simulink model "RM3_copy2copy"  (R2017b)
settings: Solver=ode4  StartTime=0  StopTime=5000  FixedStep=0.1  MaxStep=0.1  RelTol=1e-3  EnableMultiTasking=on
model workspace (MAT data in the model file):
  p1 = Simulink.Signal
  p1.DataType = 'double'
  p1.Dimensions = -1
  p1.DimensionsMode = 'auto'
  p1.Complexity = 'auto'
  p1.SampleTime = -1
  p1.SamplingMode = 'auto'
values from neighbouring files (symbols this model uses):
  m = min(Out,[],2)    [ContinousControl.m]    (also in RL.m; RealTime_modif22.m)
  N = No*n    (= 60)    [ACTOR_CRITIC & SARSA.m]    (also in TDlearningExampleEforPosting.m)
  num_act = size(action,1)    [CS533DQN_FunctionApproximation.m]    (also in ContinousControl.m; DeepQLearningF.m; HopeGreatRLCode.m; LastFixedEta.m)
  num_state = size(state_spc,1)    [CS533DQN_FunctionApproximation.m]    (also in ContinousControl.m = size(states_space,1); DeepQLearningF.m; HopeGreatRLCode.m; LastFixedEta.m)
  pnum = 1    [ContinousControl.m]    (also in RealTime_modif22.m)
  s = tf('s')    [Fe_extract.m]    (also in InputDataExtraction.m; LetsStartIt.m; SafeLetsStartIt.m; StateExtraction.m)
  states_space = states_spaceP    [ContinousControl.m]    (also in Forward_step.m = states_spaceP([1:9 6*9+1:9*7 15*9+1:9*16 5*9+1:9*6],:); RealTime_modif22.m)
  Ts = states_space( state_idx,2)    [ContinousControl.m]    (also in DeepQLearningF.m = states_space(state_idx,2); EtanStateExtraction.m = TsVec(ts); Forward_step.m = states_space( st_chosen,2); InputDataExtraction.m = TsVec(ts))
  X = YX(:,2:end)    [L2adaptivepredictor.m]
  Y = YX(:,1)    [L2adaptivepredictor.m]
undefined symbols (not defined in the file or in its folder): body, constraint, pto, Z
libraries: nesl_utility x8, sm_lib x5, WECSim_Lib x4, dspstat3 x1, dspindex x1, simulink x1
settings Model: Creator=mlawson  LastModifiedBy=ghleila
settings SolverCC: ZeroCrossControl=DisableAll  AlgebraicLoopSolver=LineSearch  AutoInsertRateTranBlk=on
settings DataIOCC: SaveFormat=Array  SaveOutput=off  SaveTime=off
settings OptimizationCC: LifeSpan=inf  SimCompilerOptimization=on
settings DebuggingCC: UnderspecifiedInitializationDetection=Classic  MergeDetectMultiDrivingBlocksExec=none  SolverPrmCheckMsg=warning  MultiTaskDSMMsg=none  AllowSymbolicDim=off  StateNameClashWarn=warning  SFUnexpectedBacktrackingDiag=warning  SFNoUnconditionalDefaultTransitionDiag=warning  SFExecutionAtInitializationDiag=none
settings HardwareCC: ProdBitPerPointer=32  ProdBitPerSizeT=32  ProdBitPerPtrDiffT=32  ProdLargestAtomicFloat=None  ProdIntDivRoundTo=Undefined  ProdEndianess=Unspecified  ProdWordSize=32  ProdHWDeviceType=32-bit Generic
settings ModelReferenceCC: PropagateSignalLabelsOutOfModel=off
settings CodeAppCC: StateflowObjectComments=on
settings GRTTargetCC: TargetLangStandard=C89/C90 (ANSI)  GeneratePreprocessorConditionals=Disable all
settings ConfigComp: CovMetricSettings=dw  CovHtmlReporting=on  CovSaveCumulativeToWorkspaceVar=on  CovSaveSingleToWorkspaceVar=on  CovExternalEMLEnable=off  CovSFcnEnable=off
settings SimscapeCC: SimscapeNormalizeSystem=off

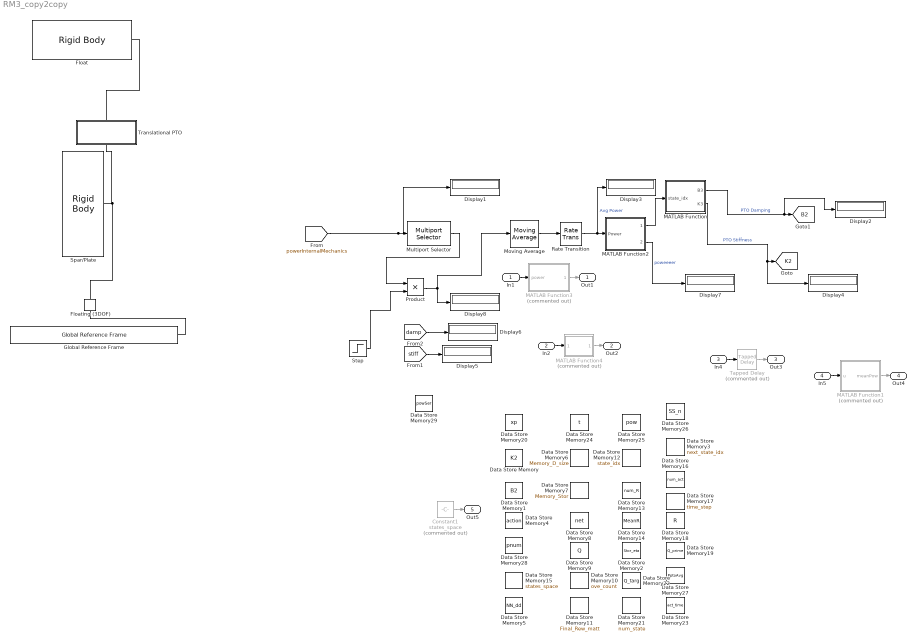
== system RM3_copy2copy ==
  In1 : Inport
  In2 : Inport  Port=2
  In4 : Inport  Port=3
  In5 : Inport  Port=4
  Constant1 : Constant  Commented=on  Value=states_space
  Data Store Memory : DataStoreMemory  DataStoreName=K2  ReadBeforeWriteMsg=warning  WriteAfterWriteMsg=warning  WriteAfterReadMsg=warning  InitialValue=K2  VectorParams1D=off  ShowAdditionalParam=off  OutDataTypeStr=double
  Data Store Memory1 : DataStoreMemory  DataStoreName=B2  ReadBeforeWriteMsg=warning  WriteAfterWriteMsg=warning  WriteAfterReadMsg=warning  InitialValue=B2  VectorParams1D=off  ShowAdditionalParam=off  OutDataTypeStr=double
  Data Store Memory10 : DataStoreMemory  DataStoreName=ove_count  ReadBeforeWriteMsg=warning  WriteAfterWriteMsg=warning  WriteAfterReadMsg=warning  InitialValue=1  VectorParams1D=off  ShowAdditionalParam=off  OutDataTypeStr=double
  Data Store Memory11 : DataStoreMemory  DataStoreName=Final_Rew_matt  ReadBeforeWriteMsg=warning  WriteAfterWriteMsg=warning  WriteAfterReadMsg=warning  InitialValue=zeros(num_state,1)  ShowAdditionalParam=off  OutDataTypeStr=double
  Data Store Memory12 : DataStoreMemory  DataStoreName=state_idx  ReadBeforeWriteMsg=warning  WriteAfterWriteMsg=warning  WriteAfterReadMsg=warning  InitialValue=state_idx  VectorParams1D=off  ShowAdditionalParam=off  OutDataTypeStr=double
  Data Store Memory13 : DataStoreMemory  DataStoreName=num_R  ReadBeforeWriteMsg=warning  WriteAfterWriteMsg=warning  WriteAfterReadMsg=warning  InitialValue=zeros(num_state,1)  VectorParams1D=off  ShowAdditionalParam=off  OutDataTypeStr=double
  Data Store Memory14 : DataStoreMemory  DataStoreName=MeanR  ReadBeforeWriteMsg=warning  WriteAfterWriteMsg=warning  WriteAfterReadMsg=warning  InitialValue=zeros(num_state,1)  VectorParams1D=off  ShowAdditionalParam=off  OutDataTypeStr=double
  Data Store Memory15 : DataStoreMemory  DataStoreName=states_space  ReadBeforeWriteMsg=warning  WriteAfterWriteMsg=warning  WriteAfterReadMsg=warning  InitialValue=states_space  VectorParams1D=off  ShowAdditionalParam=off  OutDataTypeStr=double
  Data Store Memory16 : DataStoreMemory  DataStoreName=num_act  ReadBeforeWriteMsg=warning  WriteAfterWriteMsg=warning  WriteAfterReadMsg=warning  ShowAdditionalParam=off  OutDataTypeStr=double
  Data Store Memory17 : DataStoreMemory  DataStoreName=time_step  ReadBeforeWriteMsg=warning  WriteAfterWriteMsg=warning  WriteAfterReadMsg=warning  ShowAdditionalParam=off  OutDataTypeStr=double
  Data Store Memory18 : DataStoreMemory  DataStoreName=R  ReadBeforeWriteMsg=warning  WriteAfterWriteMsg=warning  WriteAfterReadMsg=warning  InitialValue=zeros(num_state,100)  VectorParams1D=off  ShowAdditionalParam=off  OutDataTypeStr=double
  Data Store Memory19 : DataStoreMemory  DataStoreName=Q_prime  ReadBeforeWriteMsg=warning  WriteAfterWriteMsg=warning  WriteAfterReadMsg=warning  InitialValue=rand(num_state,num_act)  VectorParams1D=off  ShowAdditionalParam=off  OutDataTypeStr=double
  Data Store Memory2 : DataStoreMemory  DataStoreName=Stor_eta  ReadBeforeWriteMsg=warning  WriteAfterWriteMsg=warning  WriteAfterReadMsg=warning  InitialValue=zeros(4000,5)  VectorParams1D=off  ShowAdditionalParam=off  OutDataTypeStr=double
  Data Store Memory20 : DataStoreMemory  DataStoreName=xp  ReadBeforeWriteMsg=warning  WriteAfterWriteMsg=warning  WriteAfterReadMsg=warning  InitialValue=zeros(1,2)  VectorParams1D=off  ShowAdditionalParam=off  OutDataTypeStr=double
  Data Store Memory21 : DataStoreMemory  DataStoreName=num_state  ReadBeforeWriteMsg=warning  WriteAfterWriteMsg=warning  WriteAfterReadMsg=warning  ShowAdditionalParam=off  OutDataTypeStr=double
  Data Store Memory22 : DataStoreMemory  DataStoreName=Q_targ  ReadBeforeWriteMsg=warning  WriteAfterWriteMsg=warning  WriteAfterReadMsg=warning  InitialValue=rand(num_state,num_act)  VectorParams1D=off  ShowAdditionalParam=off  OutDataTypeStr=double
  Data Store Memory23 : DataStoreMemory  DataStoreName=act_time  ReadBeforeWriteMsg=warning  WriteAfterWriteMsg=warning  WriteAfterReadMsg=warning  ShowAdditionalParam=off  OutDataTypeStr=double
  Data Store Memory24 : DataStoreMemory  DataStoreName=t  ReadBeforeWriteMsg=warning  WriteAfterWriteMsg=warning  WriteAfterReadMsg=warning  InitialValue=1  VectorParams1D=off  ShowAdditionalParam=off  OutDataTypeStr=double
  Data Store Memory25 : DataStoreMemory  DataStoreName=pow  ReadBeforeWriteMsg=warning  WriteAfterWriteMsg=warning  WriteAfterReadMsg=warning  InitialValue=zeros(1,5100)  VectorParams1D=off  ShowAdditionalParam=off  OutDataTypeStr=double
  Data Store Memory26 : DataStoreMemory  DataStoreName=SS_n  ReadBeforeWriteMsg=warning  WriteAfterWriteMsg=warning  WriteAfterReadMsg=warning  InitialValue=SS_n  VectorParams1D=off  ShowAdditionalParam=off  OutDataTypeStr=double
  Data Store Memory27 : DataStoreMemory  DataStoreName=PptoAvg  ReadBeforeWriteMsg=warning  WriteAfterWriteMsg=warning  WriteAfterReadMsg=warning  ShowAdditionalParam=off  OutDataTypeStr=double
  Data Store Memory28 : DataStoreMemory  DataStoreName=pnum  ReadBeforeWriteMsg=warning  WriteAfterWriteMsg=warning  WriteAfterReadMsg=warning  ShowAdditionalParam=off  OutDataTypeStr=double
  Data Store Memory29 : DataStoreMemory  DataStoreName=powSer  ReadBeforeWriteMsg=warning  WriteAfterWriteMsg=warning  WriteAfterReadMsg=warning  InitialValue=zeros(1,20*Ts/0.1)  VectorParams1D=off  ShowAdditionalParam=off  OutDataTypeStr=double
  Data Store Memory3 : DataStoreMemory  DataStoreName=next_state_idx  ReadBeforeWriteMsg=warning  WriteAfterWriteMsg=warning  WriteAfterReadMsg=warning  InitialValue=1  ShowAdditionalParam=off  OutDataTypeStr=double
  Data Store Memory4 : DataStoreMemory  DataStoreName=action  ReadBeforeWriteMsg=warning  WriteAfterWriteMsg=warning  WriteAfterReadMsg=warning  InitialValue=action  VectorParams1D=off  ShowAdditionalParam=off  OutDataTypeStr=double
  Data Store Memory5 : DataStoreMemory  DataStoreName=NN_dd  ReadBeforeWriteMsg=warning  WriteAfterWriteMsg=warning  WriteAfterReadMsg=warning  InitialValue=NN_dd  ShowAdditionalParam=off  OutDataTypeStr=double
  Data Store Memory6 : DataStoreMemory  DataStoreName=Memory_D_size  ReadBeforeWriteMsg=warning  WriteAfterWriteMsg=warning  WriteAfterReadMsg=warning  InitialValue=Memory_D_size  VectorParams1D=off  ShowAdditionalParam=off  OutDataTypeStr=double
  Data Store Memory7 : DataStoreMemory  DataStoreName=Memory_Stor  ReadBeforeWriteMsg=warning  WriteAfterWriteMsg=warning  WriteAfterReadMsg=warning  InitialValue=zeros(4000,4+size(states_space,2)+num_act)  ShowAdditionalParam=off  OutDataTypeStr=double
  Data Store Memory8 : DataStoreMemory  DataStoreName=net  ReadBeforeWriteMsg=warning  WriteAfterWriteMsg=warning  WriteAfterReadMsg=warning  VectorParams1D=off  ShowAdditionalParam=off  OutDataTypeStr=double
  Data Store Memory9 : DataStoreMemory  DataStoreName=Q  ReadBeforeWriteMsg=warning  WriteAfterWriteMsg=warning  WriteAfterReadMsg=warning  InitialValue=rand(num_state,num_act)  VectorParams1D=off  ShowAdditionalParam=off  OutDataTypeStr=double
  Display{1..8} (8 alike) : Display
  Float : WECSim_Lib/Body Elements/Rigid Body  body=body(1)
      settings: AttributesFormatString=%<body>
  Floating (3DOF) : WECSim_Lib/Constraints/Floating (3DOF)  constraint=constraint(1)
      settings: AttributesFormatString=%<constraint>
  Global Reference Frame : WECSim_Lib/Frames/Global Reference Frame  waves=waves  simu=simu
  MATLAB Function : MATLAB Function  TreatAsAtomicUnit=on
  MATLAB Function1 : MATLAB Function  Commented=on  TreatAsAtomicUnit=on
  MATLAB Function2 : MATLAB Function  TreatAsAtomicUnit=on
  MATLAB Function3 : MATLAB Function  Commented=on  TreatAsAtomicUnit=on
  MATLAB Function4 : MATLAB Function  Commented=on  TreatAsAtomicUnit=on
  Moving Average : dspstat3/Moving Average  Method=Sliding window  SpecifyWindowLength=on  WindowLength=20*Ts/0.1  ForgettingFactor=0.9  SimulateUsing=Code generation
  Multiport Selector : dspindex/Multiport Selector  rowsOrCols=Rows  idxCellArray={ 3}  idxErrMode=Clip Index
  Product : Product
  Rate Transition : RateTransition  OutPortSampleTime=20*Ts
  Spar/Plate : WECSim_Lib/Body Elements/Rigid Body  body=body(2)
      settings: AttributesFormatString=%<body>
  Step : Step  SampleTime=20*pnum*10
  Tapped Delay : simulink/Discrete/Tapped Delay  Commented=on  vinit=0.0  samptime=-1  NumDelays=4  DelayOrder=Oldest  includeCurrent=off
  Translational PTO : Subsystem  AncestorBlock=WECSim_Lib/PTOs/Translational PTO  mask(PTO){pto=pto(1)}
      mask prompts: pto "PTO Name:"
      mask help:
      | Constraints the follower to translational motion relative to the base, in
      | the PTO's Z-direction and adds PTO stiffness and damping.
      |
      |
      | The variable name input below must be 'pto(i)' where i=1,2,...
      | pto(i) must be defined in the input file with the following fields:
      |
      |     .name (required)
      |             String.
      |             PTO name. Must comply with Matlab's variable naming rules.
      |     .loc (optional)
      |             3x1 vector [x y z] in meters.
      |             PTO location. Default = [0 0 0]
      |     .k (optional)
      |             Float.
      |             PTO linear spring stiffness. Default = 0
      |     .c (optional)
      |             Float.
      |             PTO linear damping coefficient. Default = 0
      |     .orientation.z (optional)
      |             3x1 vector [x y z].
      |             Direction of the PTO's Z-coordinate. Default = [0 0 1]
      |     .orientation.y (optional)
      |             3x1 vector [x y z].
      |             Direction of the PTO's Y-coordinate. Default = [0 1 0]
      mask init:
      | if exist('pto','var')
      |     h=[gcb '/output'];
      |     responseName=['pto' num2str(pto.ptoNum) '_out'];
      |     set_param(h,'VariableName',responseName);
      | end
      | 
      | pto.checkLoc('W');
      settings: AttributesFormatString=%<pto>
      mask Help:
      | Constraints the follower to translational motion relative to the base, in
      | the PTO's Z-direction and adds PTO stiffness and damping.
      | 
      | 
      | The variable name input below must be 'pto(i)' where i=1,2,...
      | pto(i) must be defined in the input file with the following fields:
      | 
      |     .name (required)
      |             String.
      |             PTO name. Must comply with Matlab's variable naming rules.
      |     .loc (optional)
      |             3x1 vector [x y z] in meters.
      |             PTO location. Default = [0 0 0]
      |     .k (optional)
      |             Float.
      |             PTO linear spring stiffness. Default = 0
      |     .c (optional)
      |             Float.
      |             PTO linear damping coefficient. Default = 0
      |     .orientation.z (optional)
      |             3x1 vector [x y z].
      |             Direction of the PTO's Z-coordinate. Default = [0 0 1]
      |     .orientation.y (optional)
      |             3x1 vector [x y z].
      |             Direction of the PTO's Y-coordinate. Default = [0 1 0]
  Out1 : Outport
  Out2 : Outport  Port=2
  Out3 : Outport  Port=3
  Out4 : Outport  Port=4
  Out5 : Outport  Port=5
  tag scope: B2=global, K2=global
  wires:
  In4/1 -> Tapped Delay/1
  MATLAB Function4/1(powSer1) -> Out2/1
  In2/1 -> MATLAB Function4/1(WholepowSer)
  MATLAB Function/1(B3) -> Display2/1, [B2]  "PTO Damping"
  [damp] -> Display6/1
  In5/1 -> MATLAB Function1/1(u)
  Tapped Delay/1 -> Out3/1
  Multiport Selector/1 -> Product/1
  MATLAB Function2/1(state_idx1) -> MATLAB Function/1(state_idx)
  Step/1 -> Product/2
  [stiff] -> Display5/1
  Moving Average/1 -> Rate Transition/1
  Constant1/1 -> Out5/1
  MATLAB Function3/1(PowSum) -> Out1/1
  MATLAB Function1/1(meanPow) -> Out4/1
  In1/1 -> MATLAB Function3/1(power)
  [powerInternalMechanics] -> Display1/1, Multiport Selector/1
  MATLAB Function/2(K3) -> Display4/1, [K2]  "PTO Stiffness"
  Rate Transition/1 -> Display3/1, MATLAB Function2/1(Power)  "Avg Power"
  Product/1 -> Display8/1, Moving Average/1
  MATLAB Function2/2(PptoAvg1) -> Display7/1  "poweeeer"
  connections:
  Translational PTO/RConn1 -- Floating (3DOF)/RConn1 -- Spar/Plate/RConn1
  Floating (3DOF)/LConn1 -- Global Reference Frame/RConn1
  Translational PTO/LConn1 -- Float/RConn1

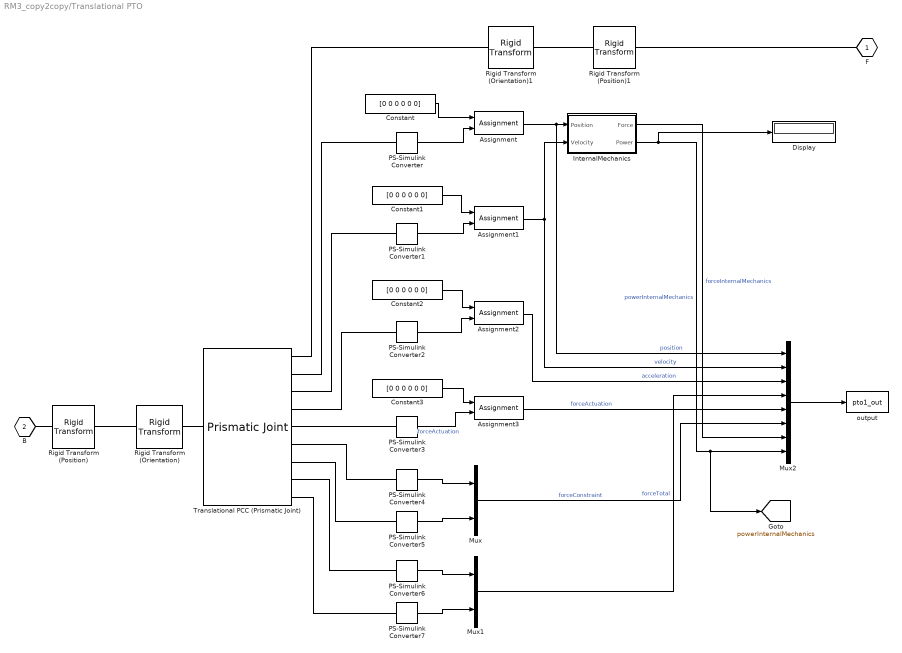
== system RM3_copy2copy/Translational PTO ==
  Assignment{,1..3} (4 alike) : Assignment  IndexOptions=Index vector (dialog)  Indices=3  OutputSizes=1
  Constant{,1..3} (4 alike) : Constant  Value=[0 0 0 0 0 0]
  Display : Display
  InternalMechanics : Subsystem
  Mux : Mux  Inputs=2
  Mux1 : Mux  Inputs=2
  Mux2 : Mux  Inputs=8
  PS-Simulink Converter{,1..7} (8 alike) : nesl_utility/PS-Simulink Converter  PhysicalDomain=network_engine_domain  SubClassName=ps_output  LeftPortType=input  RightPortType=output  PseudoPeriodic=off  Frequencies=[]  Unit=1  AffineConversion=off
  Rigid Transform (Position) : sm_lib/Frames and Transforms/Rigid Transform  TranslationMethod=Cartesian  TranslationStandardOffset=0  TranslationLengthUnit=m  TranslationStandardAxis=+Z  TranslationCartesianOffset=pto.initDisp.initLinDisp + pto.loc  TranslationROffset=0  TranslationROffsetUnits=m  TranslationZOffset=0  TranslationZOffsetUnits=m  TranslationThetaOffset=0  TranslationThetaOffsetUnits=deg  RotationMethod=None  RotationAngleUnits=rad  RotationStandardAxis=+Y  RotationAngle=0  RotationArbitraryAxis=[0 1 0]  FollAlignAxisA=+X  BaseAlignAxisA=+Y  FollAlignAxisB=+Y  BaseAlignAxisB=+Z  RotationSequenceAxes=FollowerAxes  RotationSequence=XYX  RotationSequenceAngles=[0 0 0]  RotationSequenceAnglesUnits=deg  RotationMatrix=[1 0 0; 0 1 0; 0 0 1]
  Rigid Transform (Position)1 : sm_lib/Frames and Transforms/Rigid Transform  TranslationMethod=Cartesian  TranslationStandardOffset=0  TranslationLengthUnit=m  TranslationStandardAxis=+Z  TranslationCartesianOffset=pto.initDisp.initLinDisp + pto.loc  TranslationROffset=0  TranslationROffsetUnits=m  TranslationZOffset=0  TranslationZOffsetUnits=m  TranslationThetaOffset=0  TranslationThetaOffsetUnits=deg  RotationMethod=None  RotationAngleUnits=rad  RotationStandardAxis=+Y  RotationAngle=0  RotationArbitraryAxis=[0 1 0]  FollAlignAxisA=+X  BaseAlignAxisA=+Y  FollAlignAxisB=+Y  BaseAlignAxisB=+Z  RotationSequenceAxes=FollowerAxes  RotationSequence=XYX  RotationSequenceAngles=[0 0 0]  RotationSequenceAnglesUnits=deg  RotationMatrix=[1 0 0; 0 1 0; 0 0 1]
  Rigid Transform (Orientation) : sm_lib/Frames and Transforms/Rigid Transform  TranslationMethod=None  TranslationStandardOffset=0  TranslationLengthUnit=m  TranslationStandardAxis=+Z  TranslationCartesianOffset=0  TranslationROffset=0  TranslationROffsetUnits=m  TranslationZOffset=0  TranslationZOffsetUnits=m  TranslationThetaOffset=0  TranslationThetaOffsetUnits=deg  RotationMethod=RotationMatrix  RotationAngleUnits=rad  RotationStandardAxis=+Y  RotationAngle=0  RotationArbitraryAxis=[0 1 0]  FollAlignAxisA=+X  BaseAlignAxisA=+Y  FollAlignAxisB=+Y  BaseAlignAxisB=+Z  RotationSequenceAxes=FollowerAxes  RotationSequence=XYX  RotationSequenceAngles=[0 0 0]  RotationSequenceAnglesUnits=deg  RotationMatrix=pto.orientation.rotationMatrix
  Rigid Transform (Orientation)1 : sm_lib/Frames and Transforms/Rigid Transform  TranslationMethod=None  TranslationStandardOffset=0  TranslationLengthUnit=m  TranslationStandardAxis=+Z  TranslationCartesianOffset=0  TranslationROffset=0  TranslationROffsetUnits=m  TranslationZOffset=0  TranslationZOffsetUnits=m  TranslationThetaOffset=0  TranslationThetaOffsetUnits=deg  RotationMethod=RotationMatrix  RotationAngleUnits=rad  RotationStandardAxis=+Y  RotationAngle=0  RotationArbitraryAxis=[0 1 0]  FollAlignAxisA=+X  BaseAlignAxisA=+Y  FollAlignAxisB=+Y  BaseAlignAxisB=+Z  RotationSequenceAxes=FollowerAxes  RotationSequence=XYX  RotationSequenceAngles=[0 0 0]  RotationSequenceAnglesUnits=deg  RotationMatrix=pto.orientation.rotationMatrix
  Translational PCC (Prismatic Joint) : sm_lib/Joints/Prismatic Joint  SenseConstraintForce=on  SenseConstraintForceX=off  SenseConstraintForceY=off  SenseConstraintForceZ=off  SenseConstraintTorque=on  SenseConstraintTorqueX=off  SenseConstraintTorqueY=off  SenseConstraintTorqueZ=off  SenseTotalForce=on  SenseTotalForceX=off  SenseTotalForceY=off  SenseTotalForceZ=off  SenseTotalTorque=on  SenseTotalTorqueX=off  SenseTotalTorqueY=off  SenseTotalTorqueZ=off  CompositeWrenchDir=BaseOnFollower  CompositeWrenchFrame=BaseFrame  EquilibriumPosition=0  EquilibriumPositionUnits=m  SpringStiffness=pto.k  SpringStiffnessUnits=N/m  DampingCoefficient=pto.c  DampingCoefficientUnits=N/(m/s)  TorqueActuationMode=NoTorque  MotionActuationMode=ComputedMotion  SensePosition=on  SenseVelocity=on  SenseAcceleration=on  SenseTorqueForce=on  PositionTargetSpecify=off  PositionTargetPriority=High  PositionTargetValue=0  PositionTargetValueUnits=m  VelocityTargetSpecify=off  VelocityTargetPriority=High  VelocityTargetValue=0  VelocityTargetValueUnits=m/s
  output : ToWorkspace  VariableName=pto1_out  SaveFormat=Structure With Time  SampleTime=-1
      settings: Decimation=round(simu.dtOut/simu.dt,0)
  F : PMIOPort  Port=1  Side=Left
  B : PMIOPort  Port=2  Side=Right
  tag scope: powerInternalMechanics=global
  wires:
  PS-Simulink Converter3/1 -> Assignment3/2  "forceActuation"
  Constant3/1 -> Assignment3/1
  InternalMechanics/2(Power) -> Display/1, [powerInternalMechanics], Mux2/8  "powerInternalMechanics"
  InternalMechanics/1(Force) -> Mux2/7  "forceInternalMechanics"
  PS-Simulink Converter2/1 -> Assignment2/2
  Constant2/1 -> Assignment2/1
  PS-Simulink Converter1/1 -> Assignment1/2
  Constant1/1 -> Assignment1/1
  PS-Simulink Converter/1 -> Assignment/2
  Constant/1 -> Assignment/1
  Assignment2/1 -> Mux2/3  "acceleration"
  Assignment1/1 -> InternalMechanics/2(Velocity), Mux2/2  "velocity"
  Assignment/1 -> InternalMechanics/1(Position), Mux2/1  "position"
  Assignment3/1 -> Mux2/5  "forceActuation"
  PS-Simulink Converter7/1 -> Mux1/2
  PS-Simulink Converter6/1 -> Mux1/1
  PS-Simulink Converter5/1 -> Mux/2
  PS-Simulink Converter4/1 -> Mux/1
  Mux1/1 -> Mux2/4  "forceTotal"
  Mux/1 -> Mux2/6  "forceConstraint"
  Mux2/1 -> output/1
  connections:
  Rigid Transform (Position)/RConn1 -- Rigid Transform (Orientation)/LConn1
  Rigid Transform (Position)1/RConn1 -- Rigid Transform (Orientation)1/LConn1
  Rigid Transform (Orientation)/RConn1 -- Translational PCC (Prismatic Joint)/LConn1
  Translational PCC (Prismatic Joint)/RConn6 -- PS-Simulink Converter4/LConn1
  Translational PCC (Prismatic Joint)/RConn2 -- PS-Simulink Converter/LConn1
  Translational PCC (Prismatic Joint)/RConn8 -- PS-Simulink Converter6/LConn1
  Rigid Transform (Position)1/LConn1 -- F/RConn1
  Translational PCC (Prismatic Joint)/RConn3 -- PS-Simulink Converter1/LConn1
  Translational PCC (Prismatic Joint)/RConn7 -- PS-Simulink Converter5/LConn1
  Translational PCC (Prismatic Joint)/RConn4 -- PS-Simulink Converter2/LConn1
  Rigid Transform (Orientation)1/RConn1 -- Translational PCC (Prismatic Joint)/RConn1
  Translational PCC (Prismatic Joint)/RConn9 -- PS-Simulink Converter7/LConn1
  Translational PCC (Prismatic Joint)/RConn5 -- PS-Simulink Converter3/LConn1
  Rigid Transform (Position)/LConn1 -- B/RConn1

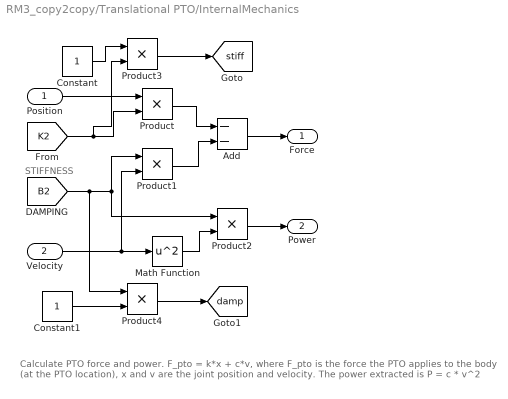
== system RM3_copy2copy/Translational PTO/InternalMechanics ==
  note: STIFFNESS
  note: Calculate PTO force and power.
      |
      | F_pto  = k*x + c*v,
      | where F_pto is the force the PTO applies to the body (at the PTO location), x and v are the joint position and velocity.
      |
      | The power extracted is
      | P = c * v^2
  Position : Inport
  Velocity : Inport  Port=2
  Add : Sum  Inputs=--
  Constant : Constant
  Constant1 : Constant
  Math Function : Math  Operator=square  SaturateOnIntegerOverflow=on
  Product{,1..4} (5 alike) : Product  Inputs=**
  Force : Outport
  Power : Outport  Port=2
  tag scope: damp=global, stiff=global
  wires:
  Product1/1 -> Add/2
  Product/1 -> Add/1
  Math Function/1 -> Product2/2
  Add/1 -> Force/1
  Position/1 -> Product/1
  [K2] -> Product3/2, Product/2
  Velocity/1 -> Product1/2, Math Function/1
  Product2/1 -> Power/1
  [B2] -> Product4/1, Product1/1, Product2/1
  Constant/1 -> Product3/1
  Product3/1 -> [stiff]
  Constant1/1 -> Product4/2
  Product4/1 -> [damp]

== matlab function RM3_copy2copy/MATLAB Function ==
  data: ove_count data_store_memory; action data_store_memory; xp data_store_memory; B2 data_store_memory; K2 data_store_memory; Stor_eta data_store_memory; states_space data_store_memory; num_R data_store_memory; MeanR data_store_memory; R data_store_memory; Final_Rew_matt data_store_memory; NN_dd data_store_memory; Memory_D_size data_store_memory; Memory_Stor data_store_memory; Q_prime data_store_memory; Q_targ data_store_memory; Q data_store_memory; B3 output; K3 output; SS_n data_store_memory; state_idx input; next_state_idx data_store_memory
function [B3,K3]=fcn1(state_idx)

global ove_count action B2 K2 Stor_eta Q states_space next_state_idx 
%B2 K2 act_time  SS_n  NN_dd Memory_D_size Memory_Stor  Q ove_count...
 %     state_idx  states_space action Stor_eta num_R MeanR  Q_targ num_state num_act time_step Q_prime  R Final_Rew_matt;


%  pow=power(end-act_time/time_step:end);
% 
% mean_six_pow=mean(pow);
%PptoAvg=mean_six_pow;





%% initial state
    
   % for ove_count1=1:1500
  
        coder.extrinsic('num2str','datasample','get_param','feedforwardnet','train'); 
        
      
   
        disp(['iteration: ' num2str(ove_count)]);
        
        %     if ove_count>=500
        %
        %          gamma=gamma_int/((ove_count)^-0.06);
        %     else
        %
        %         gamma=gamma_int;
        %
        %     end
         
          if ove_count>=150
            
            epsilon=0;
           % opts.StepRatio = 0.01;
               
                else  
            
            epsilon=1;
           % opts.StepRatio = 0.1;
            
        end
        
        %% taking an action
        
            r=rand; % get 1 uniform random number
        
            x=sum(r>=cumsum([0, 1-epsilon, epsilon])); % check it to be in which probability area
            % choose either explore or exploit
        
            if x == 1   % exploit
        
                [~,umax]=max(Q(state_idx,:));
        
                % [~,umax]=max(V(state_idx,1));
        
                current_action = action(umax,:);
        
            else        % explore
        

      % action_idx=zeros(1,1); 
        
        current_action=datasample(action,1); % choose 1 action randomly (uniform random distribution)
            end

       B2=current_action(1,1);
%        
         K2=current_action(1,2);
         
         action_idx = find(action(:,1)==B2 & action(:,2)==K2); % id of the chosen action
%         
       %         %% storing eta for reconstruction 
%         
       
Stor_eta(ove_count,1)=state_idx;
%         %Stor_eta(ove_count,2)=irreg_eta_idx

%[d f]=size(int(action_idx))
action_idx=action_idx(1,1);
        
      Stor_eta(ove_count,2)=action_idx;
      
      %% next state
        st_chosen=double(0); 
        st_chosen=datasample(1:size(states_space,1),1); % choose 1 action randomly (uniform random distribution)

        Height =states_space( st_chosen,1);           %m         %Amplitude of the waves
       
        Ts =states_space( st_chosen,2);             %s         %Significant period of the Wave

        next_state_idx1=0;
      next_state_idx1=find(states_space(:,1)==Height & states_space(:,2)==Ts & states_space(:,3)==B2 & states_space(:,4)==K2);
       next_state_idx=next_state_idx1(1,1);

gh=next_state_idx
        
        %% produce eta for the current state
        
% %         tsim_ove=60*Ts;  %%
% %         delta_t=0.01;
% %         StepT_SIM=0.01;

        %% next_state
%         
%         Height =states_space( state_idx,1);           %m         %Amplitude of the waves
%         
%         Ts =states_space( state_idx,2);
%         
%         next_stPrimee_idx=find(states_space(:,1)==Height & states_space(:,2)==Ts & states_space(:,3)==B2 & states_space(:,4)==K2);
% 
% 
%         
% % %         FeWithTime=[];
% % %         
% % %         FeWithTime=makeEtaFe(Height,Ts,tsim_ove,delta_t,A1,B1,K1);
% % %         
% % %         [PptoAvg]=TstSimulatorF(FeWithTime,A1,B1,K1,B2,K2,tsim_ove,StepT_SIM,state_idx);   % initiaL STATE
% % %       
% % %         wecSimInputFile;
% % %         wecSim;
% % %        %%% userDefinedFunctions
% % %         PP=output.ptos.powerInternalMechanics;
% % %         
% % %         mean_six_pow=mean(PP);
% % %         PptoAvg=mean_six_pow(1,3)
% % %         
% % %         hg(ove_count1)=PptoAvg;
% 
%         %% next state
%         st_chosen=double(0); 
%         st_chosen=datasample(1:size(states_space,1),1); % choose 1 action randomly (uniform random distribution)
%         
%         
%         Height_prime =states_space( st_chosen,1);           %m         %Amplitude of the waves
%         Ts_prime =states_space( st_chosen,2);             %s         %Significant period of the Wave
%         
%         next_state_idx=find(states_space(:,1)==Height_prime & states_space(:,2)==Ts_prime & states_space(:,3)==B2 & states_space(:,4)==K2);
%         
%         
%         %% allocating power
%         num_R(next_stPrimee_idx)=num_R(next_stPrimee_idx)+1;
%         next_reward=(PptoAvg/(Height^2)); %% normalized reward
%         %num_R(state_idx)=2;
%         R(next_stPrimee_idx,num_R(next_stPrimee_idx))=next_reward
%         Height=states_space(next_stPrimee_idx,1);
%         Height=Height(1,1);
%         next_state_idx;
%         
%         Period=states_space(next_stPrimee_idx,2);
%         Period=Period(1,1);
%         
%        
%         R_idx=find(states_space(:,1)==Height& states_space(:,2)==Period);
%         
%         MeanR(R_idx,1)=sum(R(R_idx,:),2)./num_R(R_idx) % mean
%         
%         % MaxR=max(max(R(R_idx)));
%         
%         MaxR=max(MeanR(R_idx));
%         
%                
%         Final_Rew_matt(R_idx)=MeanR(R_idx,1)/MaxR;
%         
%         Final_Rew=Final_Rew_matt(next_stPrimee_idx);
%         
%         Final_Rew=(Final_Rew)^5;
%         
% % %         if (PptoAvg/1e06)<=0.1
% % %             Final_Rew=-1;
% % %         end
%         
%         %     if ove_count>150
%         %
%         %         if Final_Rew==1
%         %         Final_Rew=10;
%         %         end
%         %     end
%         
%        % Stor_eta(ove_count,3)=(All_params3(1,1)); Stor_eta(ove_count,4)=(All_params3(1,2)); 
%        %%% so what
%         Stor_eta(ove_count,3)=B2;
%         Stor_eta(ove_count,4)=K2;  Stor_eta(ove_count,5)=PptoAvg;
% %         
%         
%    
%         %% storing features
%         
%        % All_features(ove_count,:)=All_params3;  %%% to get an idea about the max of each parameter
%         
%         disp(['current state : ' num2str(state_idx) ' next state : ' num2str(next_state_idx) ' taken action : ' num2str(action(action_idx,:))]);
%         
%         disp([' next reward : ' num2str(Final_Rew)]);
%         
%         %% neural network part
%         
%         
%         if ove_count> 10  %% start traing network
%             
%                         %% droping off very old data
%             
%             if ove_count>Memory_D_size %% dropoff
%                 
%                 In=Memory_Stor(ove_count-Memory_D_size:ove_count-1,5:8);
%                 
%                 Output=Memory_Stor(ove_count-Memory_D_size:ove_count-1,9:end);
%                 
%                 nodes = [size(In,2) size(action,1)];
%                 
%             else
%                 
%                 In=Memory_Stor(1:ove_count-1,5:8);
%                 
%                 Output=Memory_Stor(1:ove_count-1,9:end);
%                 
%                 nodes = [size(In,2) size(action,1)];
%                 
%             end
%             
%            % % % % %             
% % % % %             In=Memory_Stor(:,5:8);
% % % % %             
% % % % %             Output=Memory_Stor(:,9:end);
% % % % %             
%             
%                 Out=[];
%                 Out=Output;
%                 m = min(Out,[],2);  
%                 range = max(Out,[],2) - m;      
%                Out1=bsxfun(@minus,Out,m);
%                Out=bsxfun(@rdivide,Out1,range) ;
%             
%                 Input=[];
%                 Input=In;
%                 m11 = min(Input);
%                range1 = max(Input) - m11;
%                Input=bsxfun(@minus,Input,m11);
%                Input=bsxfun(@rdivide,Input,range1) ;
%                
%            
%                %% correction for one sea state
%                 Input(:,1:2) =ones(size(Input,1),2);
%             
%             net = feedforwardnet([5]);
%             [net,tr] = train(net,Input',Out');
% %             
% %             
%             y_prime= net(SS_n(next_state_idx,:)');
%             Q_prime(next_state_idx,:) =y_prime';
%             
%             
%         
%             
%             
% %             % % % %
% % % dnn=[];
% % %                 [dnn,out_est,rmse]=DNNf(Input,Output,nodes,opts);
% % %             Input;
% % %                 g=v2h(dnn, SS_n(next_state_idx,:));
% % %             
% % %                Q_prime(next_state_idx,:) = v2h(dnn, SS_n(next_state_idx,:));
% 
% %ghk=Final_Rew+gamma*max(Q_prime(next_state_idx,:)); % update q values
%            
%             sec_part=Q_prime(next_state_idx,:);
%             sec_part=sec_part(1,:);
%             ghk=Final_Rew+gamma*max(sec_part);
%             ghk=ghk(1,1);
%            Q_targ(state_idx,action_idx)=ghk; % update q values
%             
%             target=Q;
%             Q_prev=Q;
%             
%             target(state_idx,action_idx)=Q_targ(state_idx,action_idx); %%% update target
%             Memory_Stor(ove_count,:)=[state_idx,action_idx,Final_Rew,next_state_idx,states_space(state_idx,:),target(state_idx,:)];
% result=[state_idx,action_idx,Final_Rew]
%             %% training NN with recent data
%             %        [dnn,out_est,rmse]=DNNf(Input,Output,nodes,opts);
%             
%           else
%             % Q_prev=Q;
%             
%            % Q(state_idx,action_idx)=Q(state_idx,action_idx)+alpha*(Final_Rew+gamma*max(Q(next_state_idx,:))-Q(state_idx,action_idx));
%            gh=Q(next_state_idx,:);
%            MaxQ=max(gh(1,:));
%             QQ=Q(state_idx,action_idx);
%             Q3=gamma*MaxQ-Q(state_idx,action_idx);
%             Q_final=Q(state_idx,action_idx)+alpha*(Final_Rew+Q3);
%             Q(state_idx,action_idx)=Q_final(1,1);
%           %  Q(state_idx,action_idx)=Q(state_idx,action_idx)+alpha*(Final_Rew+gamma*max(Q(next_state_idx,:))-Q(state_idx,action_idx));
%             target=Q;
%             
%             Memory_Stor(ove_count,:)=[state_idx,action_idx,Final_Rew,next_state_idx,states_space(state_idx,:),target(state_idx,:)];
%         end
%         
%         %% checking the convergence of  Q function
%         
%         Q=target;
%         
%         % dif(ove_count)=norm(target(:,:)-Q_prev(:,:),Inf);
%         
%         ove_count=ove_count+1;
%         next_state_idx=next_state_idx(1,1);
%         
%         state_idx=next_state_idx;
%         
%    % end
        

B3=B2
K3=K2
        h=1;
        
        
       % d=xp(1,2)

== matlab function RM3_copy2copy/MATLAB Function1 ==
  settings: updateMethod=DISCRETE
  data: u input; t data_store_memory; pow data_store_memory; meanPow output
function meanPow=fcn(u)

%codegen

global t pow
%coder.varsize('k',[1 5000]);

 coder.extrinsic('average')
 k=zeros(1,t);
          pow(1,t)=u(3,:);
          k=pow(1,1:t);
          meanPow=0;
          meanPow=mean(k(1,:));
  
          t=t+1;
%         PptoAvg=mean_six_pow(1,3);

== matlab function RM3_copy2copy/MATLAB Function2 ==
  data: ove_count data_store_memory; action data_store_memory; xp data_store_memory; B2 data_store_memory; K2 data_store_memory; Stor_eta data_store_memory; state_idx data_store_memory; states_space data_store_memory; num_R data_store_memory; MeanR data_store_memory; R data_store_memory; Final_Rew_matt data_store_memory; NN_dd data_store_memory; Memory_D_size data_store_memory; Memory_Stor data_store_memory; Q_prime data_store_memory; Q_targ data_store_memory; Q data_store_memory; Power input; state_idx1 output; SS_n data_store_memory; next_state_idx data_store_memory; PptoAvg data_store_memory; PptoAvg1 output; pnum data_store_memory
function [state_idx1,PptoAvg1] =fcn1(Power)

global ove_count action B2 K2 Stor_eta states_space num_R MeanR state_idx R Final_Rew_matt...
    NN_dd Memory_D_size Memory_Stor Q_prime Q_targ Q SS_n next_state_idx PptoAvg pnum
%B2 K2 act_time  SS_n  NN_dd Memory_D_size Memory_Stor  Q ove_count...
%     state_idx  states_space action Stor_eta num_R MeanR  Q_targ num_state num_act time_step Q_prime  R Final_Rew_matt;


pnum=pnum+1; %set the p1 to zero for next iters

Ts=10; %%% should be global
num=20*Ts/0.1;  %% should be global
%Power=Power/num;

%PptoAvg=Power-PptoAvg;
PptoAvg=Power;

PptoAvg1=PptoAvg;

%  pow=power(end-act_time/time_step:end);
%
% mean_six_pow=mean(pow);
%PptoAvg=mean_six_pow;
%% initial state

% for ove_count1=1:1500

coder.extrinsic('num2str','datasample','get_param','feedforwardnet','train');


if ove_count>=150
    
    gamma=0.9;
    % opts.StepRatio = 0.01;
else
    
    gamma=0.6;
    % opts.StepRatio = 0.1;
    
end


if ove_count>=150
    
    alpha=0.6;
    
else
    
    alpha=0.4;
    
end




%         %% taking an action
%
%             r=rand; % get 1 uniform random number
%
%             x=sum(r>=cumsum([0, 1-epsilon, epsilon])); % check it to be in which probability area
%             % choose either explore or exploit
%
%             if x == 1   % exploit
%
%                 [~,umax]=max(Q(state_idx,:));
%
%                 % [~,umax]=max(V(state_idx,1));
%
%                 current_action = action(umax,:);
%
%             else        % explore
%
%
%       % action_idx=zeros(1,1);
%
%         current_action=datasample(action,1); % choose 1 action randomly (uniform random distribution)
%             end
%
%        B2=current_action(1,1);
% %
%          K2=current_action(1,2);
%
%          action_idx = find(action(:,1)==B2 & action(:,2)==K2); % id of the chosen action
% %
%        %         %% storing eta for reconstruction
% %
%
% Stor_eta(ove_count,1)=state_idx;
% %         %Stor_eta(ove_count,2)=irreg_eta_idx
%
% %[d f]=size(int(action_idx))
% action_idx=action_idx(1,1);
%
%       Stor_eta(ove_count,2)=action_idx;
%
%% produce eta for the current state

% %         tsim_ove=60*Ts;  %%
% %         delta_t=0.01;
% %         StepT_SIM=0.01;

%% next_state



action_idx = find(action(:,1)==B2 & action(:,2)==K2);

Height =states_space( next_state_idx,1);           %m         %Amplitude of the waves

Ts =states_space( next_state_idx,2);

% next_stPrimee_idx=find(states_space(:,1)==Height & states_space(:,2)==Ts & states_space(:,3)==B2 & states_space(:,4)==K2);



% %         FeWithTime=[];
% %
% %         FeWithTime=makeEtaFe(Height,Ts,tsim_ove,delta_t,A1,B1,K1);
% %
% %         [PptoAvg]=TstSimulatorF(FeWithTime,A1,B1,K1,B2,K2,tsim_ove,StepT_SIM,state_idx);   % initiaL STATE
% %
% %         wecSimInputFile;
% %         wecSim;
% %        %%% userDefinedFunctions
% %         PP=output.ptos.powerInternalMechanics;
% %
% %         mean_six_pow=mean(PP);
% %         PptoAvg=mean_six_pow(1,3)
% %
% %         hg(ove_count1)=PptoAvg;

%% next state
%         st_chosen=double(0);
%         st_chosen=datasample(1:size(states_space,1),1); % choose 1 action randomly (uniform random distribution)
%
%
%         Height_prime =states_space( st_chosen,1);           %m         %Amplitude of the waves
%         Ts_prime =states_space( st_chosen,2);             %s         %Significant period of the Wave
%
%         next_state_idx=find(states_space(:,1)==Height_prime & states_space(:,2)==Ts_prime & states_space(:,3)==B2 & states_space(:,4)==K2);


%% allocating power
num_R(next_state_idx)=num_R(next_state_idx)+1;
next_reward=(PptoAvg/(Height^2)); %% normalized reward
%num_R(state_idx)=2;
%         next_state_idx
%         next_reward
R(next_state_idx,num_R(next_state_idx))=next_reward;
Height=states_space(next_state_idx,1);
Height=Height(1,1);
next_state_idx;

Period=states_space(next_state_idx,2);
Period=Period(1,1);


R_idx=find(states_space(:,1)==Height& states_space(:,2)==Period);

MeanR(R_idx,1)=sum(R(R_idx,:),2)./num_R(R_idx); % mean

% MaxR=max(max(R(R_idx)));

MaxR=max(MeanR(R_idx));


Final_Rew_matt(R_idx)=MeanR(R_idx,1)/MaxR;

Final_Rew=Final_Rew_matt(next_state_idx);

Final_Rew=(Final_Rew)^5;

% %         if (PptoAvg/1e06)<=0.1
% %             Final_Rew=-1;
% %         end

%     if ove_count>150
%
%         if Final_Rew==1
%         Final_Rew=10;
%         end
%     end

% Stor_eta(ove_count,3)=(All_params3(1,1)); Stor_eta(ove_count,4)=(All_params3(1,2));
%%% so what
Stor_eta(ove_count,3)=B2;
Stor_eta(ove_count,4)=K2;  Stor_eta(ove_count,5)=PptoAvg;
%


%% storing features

% All_features(ove_count,:)=All_params3;  %%% to get an idea about the max of each parameter

disp(['current state : ' num2str(state_idx) ' next state : ' num2str(next_state_idx) ' taken action : ' num2str(action(action_idx,:))]);

disp([' next reward : ' num2str(Final_Rew)]);

%% neural network part


if ove_count> 5  %% start traing network
    
    %% droping off very old data
    
    if ove_count>Memory_D_size %% dropoff
        
        In=Memory_Stor(ove_count-Memory_D_size:ove_count-1,5:8);
        
        Output=Memory_Stor(ove_count-Memory_D_size:ove_count-1,9:end);
        
        nodes = [size(In,2) size(action,1)];
        
    else
        
        In=Memory_Stor(1:ove_count-1,5:8);
        
        Output=Memory_Stor(1:ove_count-1,9:end);
        
        nodes = [size(In,2) size(action,1)];
        
    end
    
    % % % % %
    % % % %             In=Memory_Stor(:,5:8);
    % % % %
    % % % %             Output=Memory_Stor(:,9:end);
    % % % %
    
    Out=[];
    Out=Output;
    m = min(Out,[],2);
    range = max(Out,[],2) - m;
    Out1=bsxfun(@minus,Out,m);
    Out=bsxfun(@rdivide,Out1,range) ;
    
    Input=[];
    Input=In;
    m11 = min(Input);
    range1 = max(Input) - m11;
    Input=bsxfun(@minus,Input,m11);
    Input=bsxfun(@rdivide,Input,range1) ;
    
    
    %% correction for one sea state
    Input(:,1:2) =ones(size(Input,1),2);
    
    net = feedforwardnet([5]);
    [net,tr] = train(net,Input',Out');
    %
    %
    y_prime= net(SS_n(next_state_idx,:)');
    Q_prime(next_state_idx,:) =y_prime';
    
    
    
    
    
    %             % % % %
    % % dnn=[];
    % %                 [dnn,out_est,rmse]=DNNf(Input,Output,nodes,opts);
    % %             Input;
    % %                 g=v2h(dnn, SS_n(next_state_idx,:));
    % %
    % %                Q_prime(next_state_idx,:) = v2h(dnn, SS_n(next_state_idx,:));
    
    %ghk=Final_Rew+gamma*max(Q_prime(next_state_idx,:)); % update q values
    
    sec_part=Q_prime(next_state_idx,:);
    sec_part=sec_part(1,:);
    ghk=Final_Rew+gamma*max(sec_part);
    ghk=ghk(1,1);
    Q_targ(state_idx,action_idx)=ghk; % update q values
    
    target=Q;
    Q_prev=Q;
    
    target(state_idx,action_idx)=Q_targ(state_idx,action_idx); %%% update target
    Memory_Stor(ove_count,:)=[state_idx,action_idx,Final_Rew,next_state_idx,states_space(state_idx,:),target(state_idx,:)];
    result=[state_idx,action_idx,Final_Rew,next_state_idx]
    result2_powe=PptoAvg
    %% training NN with recent data
    %        [dnn,out_est,rmse]=DNNf(Input,Output,nodes,opts);
    
else
    % Q_prev=Q;
    
    % Q(state_idx,action_idx)=Q(state_idx,action_idx)+alpha*(Final_Rew+gamma*max(Q(next_state_idx,:))-Q(state_idx,action_idx));
    gh=Q(next_state_idx,:);
    MaxQ=max(gh(1,:));
    QQ=Q(state_idx,action_idx);
    Q3=gamma*MaxQ-Q(state_idx,action_idx);
    Q_final=Q(state_idx,action_idx)+alpha*(Final_Rew+Q3)
    Q(state_idx,action_idx)=Q_final(1,1);
    %  Q(state_idx,action_idx)=Q(state_idx,action_idx)+alpha*(Final_Rew+gamma*max(Q(next_state_idx,:))-Q(state_idx,action_idx));
    target=Q;
    
    Memory_Stor(ove_count,:)=[state_idx,action_idx,Final_Rew,next_state_idx,states_space(state_idx,:),target(state_idx,:)];
end

%% checking the convergence of  Q function

Q=target;

% dif(ove_count)=norm(target(:,:)-Q_prev(:,:),Inf);

ove_count=ove_count+1;
next_state_idx=next_state_idx(1,1);

state_idx=next_state_idx;

% end

state_idx1=state_idx;

h=1;


% d=xp(1,2)

== matlab function RM3_copy2copy/MATLAB Function3 ==
  settings: updateMethod=DISCRETE
  data: power input; PowSum output; p1 data_store_memory
function PowSum = fcn(power)

global p1
% Ts=10; %%% should be global 
% num=20*Ts/0.1;  %% should be global 

p1=p1+power(end);
PowSum=p1;
% AvgPow=1

== matlab function RM3_copy2copy/MATLAB Function4 ==
  data: WholepowSer input; powSer1 output; p1 data_store_memory; powSer data_store_memory
function powSer1 = fcn(WholepowSer)

global powSer p1

kh=WholepowSer(end);
p1=p1+1;
powSer(p1,1)=kh;

powSer1=powSer;
